simulink subsystem "StarTracker"  (R2021a)
settings: Solver=VariableStepAuto  StartTime=0.0  StopTime=10.0  RelTol=1e-3
libraries: simulink x3, aerolibutil x2, sharedutil x2, aerolibconvert2 x1
settings Model: Creator=jmher  LastModifiedBy=jmher

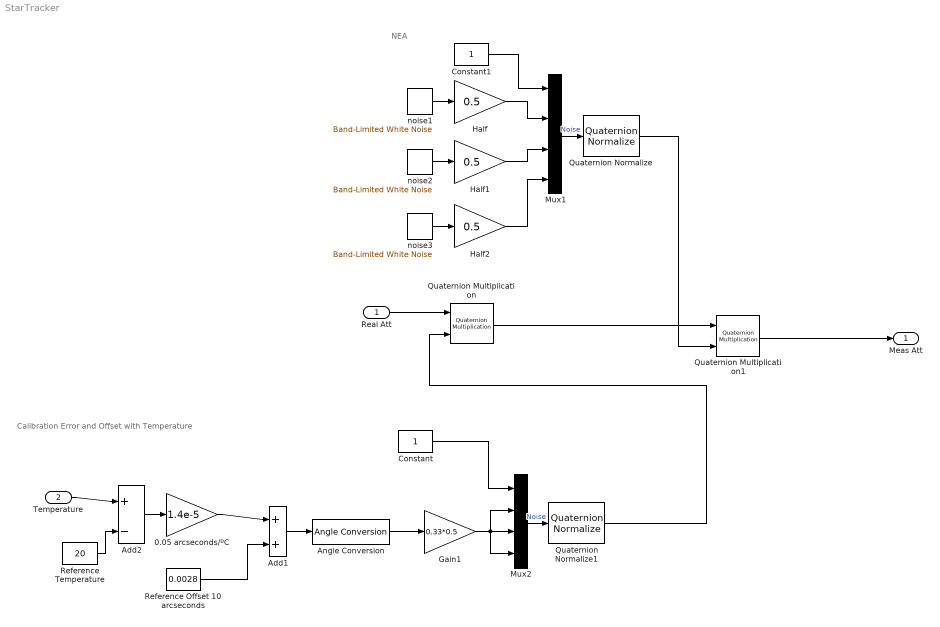
== system StarTracker ==
  note: NEA
  note: Calibration Error and Offset
      | with Temperature
  Real Att : Inport
  Temperature : Inport  Port=2
  0.05 arcseconds/ºC : Gain  Gain=1.4e-5
  Add1 : Sum  Inputs=+|+
  Add2 : Sum  Inputs=+|-
  Angle Conversion : aerolibconvert2/Angle Conversion  IU=deg  OU=rad
  Constant : Constant
  Constant1 : Constant
  Gain1 : Gain  Gain=0.33*0.5
  Half : Gain  Gain=0.5
  Half1 : Gain  Gain=0.5
  Half2 : Gain  Gain=0.5
  Mux1 : Mux
  Mux2 : Mux
  Quaternion Multiplication : aerolibutil/Quaternion Multiplication
  Quaternion Multiplication1 : aerolibutil/Quaternion Multiplication
  Quaternion Normalize : sharedutil/Quaternion Normalize  aMode=aMode
      settings: SourceProductBaseCode=AE,PW,DR,MT,UV,VE
  Quaternion Normalize1 : sharedutil/Quaternion Normalize  aMode=aMode
      settings: SourceProductBaseCode=AE,PW,DR,MT,UV,VE
  Reference Offset 10 arcseconds : Constant  Value=0.0028
  Reference Temperature : Constant  Value=20
  noise1 : simulink/Sources/Band-Limited White Noise  Cov=noiseNEA  Ts=0.01  seed=[83812]
  noise2 : simulink/Sources/Band-Limited White Noise  Cov=noiseNEA  Ts=0.01  seed=[098276]
  noise3 : simulink/Sources/Band-Limited White Noise  Cov=noiseNEA  Ts=0.01  seed=[73651]
  Meas Att : Outport
  wires:
  Quaternion Multiplication/1 -> Quaternion Multiplication1/1
  Real Att/1 -> Quaternion Multiplication/1
  Quaternion Multiplication1/1 -> Meas Att/1
  Reference Offset 10 arcseconds/1 -> Add1/2
  Add2/1 -> 0.05 arcseconds/ºC/1
  Reference Temperature/1 -> Add2/2
  Temperature/1 -> Add2/1
  0.05 arcseconds/ºC/1 -> Add1/1
  Constant1/1 -> Mux1/1
  noise1/1 -> Half/1
  noise2/1 -> Half1/1
  noise3/1 -> Half2/1
  Half1/1 -> Mux1/3
  Half2/1 -> Mux1/4
  Half/1 -> Mux1/2
  Mux1/1 -> Quaternion Normalize/1  "Noise"
  Quaternion Normalize/1 -> Quaternion Multiplication1/2
  Mux2/1 -> Quaternion Normalize1/1  "Noise"
  Quaternion Normalize1/1 -> Quaternion Multiplication/2
  Constant/1 -> Mux2/1
  Add1/1 -> Angle Conversion/1
  Gain1/1 -> Mux2/4, Mux2/2, Mux2/3
  Angle Conversion/1 -> Gain1/1
